simulink model "alba9b_full_loop"  (R2025b)
settings: Solver=ode15s  StartTime=0.0  StopTime=120  MaxStep=0.025  RelTol=2e-8  AbsTol=1e-9
undefined symbols (not defined in the file or in its folder): S_vec, V0_m3
settings Model: Creator=86155  LastModifiedBy=86155
settings DataIOCC: SaveFinalState=on  SaveOperatingPoint=on  SaveOutput=off  SaveState=on  SignalLogging=off  SaveTime=off

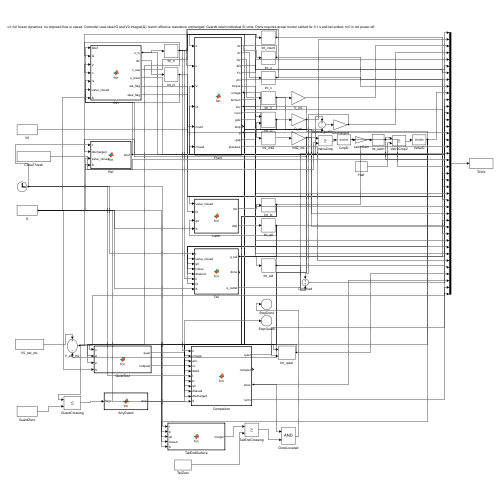
[thumbnail: Simulink's stored preview of the top-level diagram]
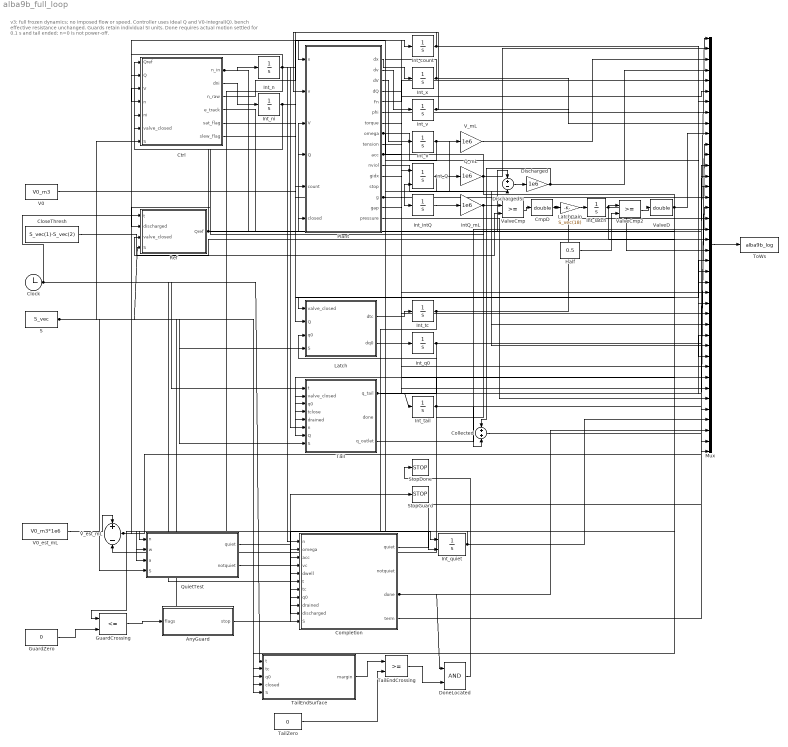
== system alba9b_full_loop ==
  note: v3: full frozen dynamics; no imposed flow or speed. Controller uses ideal Q and V0-integral(Q). bench effective resistance unchanged. Guards retain individual SI units. Done requires actual motion settled for 0.1 s and tail ended; n=0 is not power-off.
  AnyGuard : MATLAB Function  TreatAsAtomicUnit=on
  Clock : Clock
  CloseThresh : Constant  Value=S_vec(1)-S_vec(2)
  CmpD : DataTypeConversion  OutDataTypeStr=double  SaturateOnIntegerOverflow=off  RndMeth=Floor
  Collected : Sum
  Completion : MATLAB Function  TreatAsAtomicUnit=on
  Ctrl : MATLAB Function  TreatAsAtomicUnit=on
  Discharged : Gain  Gain=1e6
  DischargedSI : Sum  Inputs=+-
  DoneLocated : Logic  AllPortsSameDT=off  OutDataTypeStr=boolean
  GuardCrossing : RelationalOperator  Operator=<=  OutDataTypeStr=boolean  RndMeth=Simplest  InputSameDT=off
  GuardZero : Constant  Value=0
  Half : Constant  Value=0.5
  Int_Q : Integrator  ExternalReset=rising  AbsoluteTolerance=2e-14
  Int_V : Integrator  InitialCondition=V0_m3  AbsoluteTolerance=2e-13
  Int_count : Integrator  AbsoluteTolerance=1e-6
  Int_intQ : Integrator  AbsoluteTolerance=2e-13
  Int_latch : Integrator  LimitOutput=on  UpperSaturationLimit=1  LowerSaturationLimit=0  AbsoluteTolerance=1e-9
  Int_n : Integrator  LimitOutput=on  UpperSaturationLimit=S_vec(12)  LowerSaturationLimit=0  AbsoluteTolerance=1e-4
  Int_ni : Integrator  AbsoluteTolerance=1e-4
  Int_q0 : Integrator  AbsoluteTolerance=1e-7
  Int_quiet : Integrator  ExternalReset=rising  AbsoluteTolerance=1e-8
  Int_tail : Integrator  AbsoluteTolerance=1e-9
  Int_tc : Integrator  AbsoluteTolerance=1e-7
  Int_v : Integrator  AbsoluteTolerance=2e-10
  Int_x : Integrator  AbsoluteTolerance=2e-11
  Latch : MATLAB Function  TreatAsAtomicUnit=on
  LatchGain : Gain  Gain=S_vec(18)
  Mux : Mux  Inputs=40
  Plant : MATLAB Function  TreatAsAtomicUnit=on
  Q_mL : Gain  Gain=1e6
  QuietTest : MATLAB Function  TreatAsAtomicUnit=on
  Ref : MATLAB Function  TreatAsAtomicUnit=on
  S : Constant  Value=S_vec
  StopDone : Stop
  StopGuard : Stop
  Tail : MATLAB Function  TreatAsAtomicUnit=on
  TailEndCrossing : RelationalOperator  OutDataTypeStr=boolean  RndMeth=Simplest  InputSameDT=off
  TailEndSurface : MATLAB Function  TreatAsAtomicUnit=on
  TailZero : Constant  Value=0
  ToWs : ToWorkspace  VariableName=alba9b_log  SaveFormat=Structure With Time  SampleTime=-1
  V0 : Constant  Value=V0_m3
  V0_est_mL : Constant  Value=V0_m3*1e6
  V_est_mL : Sum  Inputs=+-
  V_mL : Gain  Gain=1e6
  ValveCmp : RelationalOperator  OutDataTypeStr=boolean  RndMeth=Simplest  InputSameDT=off
  ValveCmp2 : RelationalOperator  OutDataTypeStr=boolean  RndMeth=Simplest  InputSameDT=off
  ValveD : DataTypeConversion  OutDataTypeStr=double  SaturateOnIntegerOverflow=off  RndMeth=Floor
  intQ_mL : Gain  Gain=1e6
  wires:
  Int_x/1 -> Plant/1(x), Mux/8
  Int_v/1 -> Plant/2(v), Mux/9
  Int_V/1 -> Plant/3(V), V_mL/1, DischargedSI/2
  Int_Q/1 -> Plant/4(Q), Int_intQ/1, Q_mL/1
  Int_count/1 -> Plant/5(count), Mux/31
  ValveD/1 -> Plant/6(closed), Int_Q/2, Ref/3(valve_closed), Ctrl/6(valve_closed), Latch/1(valve_closed), Tail/2(valve_closed), Mux/10, Completion/4(vc), TailEndSurface/4(closed)
  Plant/1(dx) -> Int_x/1
  Plant/2(dv) -> Int_v/1
  Plant/3(dV) -> Int_V/1
  Plant/4(dQ) -> Int_Q/1
  Int_n/1 -> Int_count/1, Ctrl/4(n), Tail/6(n), Mux/6, Completion/1(n), QuietTest/1(n)
  Int_intQ/1 -> intQ_mL/1
  V0/1 -> DischargedSI/1
  DischargedSI/1 -> Discharged/1
  Discharged/1 -> Collected/1, Mux/4
  CloseThresh/1 -> ValveCmp/2
  ValveCmp/1 -> CmpD/1
  CmpD/1 -> LatchGain/1, Mux/21
  LatchGain/1 -> Int_latch/1
  Int_latch/1 -> ValveCmp2/1, Mux/20
  Half/1 -> ValveCmp2/2
  ValveCmp2/1 -> ValveD/1
  Clock/1 -> Ref/1(t), Tail/1(t), Completion/6(t), TailEndSurface/1(t)
  S/1 -> Ref/4(S), Ctrl/7(S), Latch/4(S), Tail/8(S), Completion/11(S), QuietTest/4(S), TailEndSurface/5(S)
  Ref/1(Qref) -> Ctrl/1(Qref), Mux/1
  Q_mL/1 -> Ctrl/2(Q), Latch/2(Q), Tail/7(Q), Mux/2
  V_mL/1 -> Mux/3
  Int_ni/1 -> Ctrl/5(ni), Mux/16
  Ctrl/1(n_in) -> Int_n/1, Mux/15
  Ctrl/2(dni) -> Int_ni/1
  Int_q0/1 -> Latch/3(q0), Tail/3(q0), Mux/17, Completion/8(q0), TailEndSurface/3(q0)
  Latch/1(dtc) -> Int_tc/1
  Latch/2(dq0) -> Int_q0/1
  Int_tc/1 -> Tail/4(tclose), Mux/18, Completion/7(tc), TailEndSurface/2(tc)
  Int_tail/1 -> Tail/5(drained), Collected/2, Mux/12, Completion/9(drained)
  Tail/1(q_tail) -> Int_tail/1, Mux/11
  Plant/5(Fn) -> Mux/5
  Ctrl/3(n_raw) -> Mux/7
  Collected/1 -> Mux/13
  Ctrl/4(e_track) -> Mux/14
  Tail/3(q_outlet) -> Mux/19
  Ctrl/5(sat_flag) -> Mux/22
  Ctrl/6(slew_flag) -> Mux/23
  Plant/6(phi) -> Mux/24
  Plant/7(torque) -> Mux/25
  Plant/8(omega) -> Mux/26, Completion/2(omega), QuietTest/2(w)
  Plant/9(tension) -> Mux/27
  Plant/11(nviol) -> Mux/28
  Plant/12(gidx) -> Mux/29
  intQ_mL/1 -> Mux/30, V_est_mL/2, Ref/2(discharged), ValveCmp/1, Completion/10(discharged)
  Plant/10(acc) -> Mux/32, Completion/3(acc), QuietTest/3(a)
  Mux/1 -> ToWs/1
  V0_est_mL/1 -> V_est_mL/1
  V_est_mL/1 -> Ctrl/3(V), Mux/36
  Int_quiet/1 -> Completion/5(dwell), Mux/37
  QuietTest/1(quiet) -> Int_quiet/1
  QuietTest/2(notquiet) -> Int_quiet/2
  TailEndSurface/1(margin) -> TailEndCrossing/1
  TailZero/1 -> TailEndCrossing/2
  Completion/3(done) -> DoneLocated/1, Mux/38
  TailEndCrossing/1 -> DoneLocated/2
  DoneLocated/1 -> StopDone/1
  Plant/14(g) -> GuardCrossing/1, Mux/33
  GuardZero/1 -> GuardCrossing/2
  GuardCrossing/1 -> AnyGuard/1(flags)
  AnyGuard/1(stop) -> StopGuard/1
  Plant/15(gap) -> Mux/34
  Plant/16(pressure) -> Mux/35
  Completion/4(term) -> Mux/39
  Completion/1(quiet) -> Mux/40

== matlab function alba9b_full_loop/Completion ==
  data: n input; quiet output; omega input; acc input; vc input; dwell input; t input; tc input; q0 input; drained input; discharged input; S input; notquiet output; done output; term output
function [quiet,notquiet,done,term] = fcn(n,omega,acc,vc,dwell,t,tc,q0,drained,discharged,S)
%#codegen
quiet=double(abs(n)<=S(22) && abs(omega)<=S(23) && abs(acc)<=S(24));
notquiet=1-quiet;
T=inf; if q0>0, T=2*S(3)/q0; end
done=double(vc>0.5 && t>=tc+T && drained>=S(3)-1e-6 && dwell>=S(25));
term=double(S(20)>0.5 && S(1)-S(2)-discharged<=S(21));
end

== matlab function alba9b_full_loop/QuietTest ==
  data: n input; quiet output; w input; a input; S input; notquiet output
function [quiet,notquiet]=fcn(n,w,a,S)
%#codegen
quiet=double(abs(n)<=S(22) && abs(w)<=S(23) && abs(a)<=S(24));
notquiet=1-quiet;
end

== matlab function alba9b_full_loop/TailEndSurface ==
  data: t input; margin output; tc input; q0 input; closed input; S input
function margin=fcn(t,tc,q0,closed,S)
%#codegen
margin=-1; if closed>0.5 && q0>0, margin=t-tc-2*S(3)/q0; end
end

== matlab function alba9b_full_loop/AnyGuard ==
  data: flags input; stop output
function stop=fcn(flags)
%#codegen
stop=any(flags);
end

== matlab function alba9b_full_loop/Ctrl ==
  data: Qref input; n_in output; Q input; V input; n input; ni input; valve_closed input; S input; dni output; n_raw output; e_track output; sat_flag output; slew_flag output
function [n_in,dni,n_raw,e_track,sat_flag,slew_flag] = fcn(Qref,Q,V,n,ni,valve_closed,S)
%#codegen
% identical to model A: same gains, same structure, no retuning in stage B
[n_in,dni,n_raw,e_track,~,sat_flag,slew_flag] = ...
    alba9_controller(Qref,Q,V,n,ni,valve_closed,S);

== matlab function alba9b_full_loop/Ref ==
  data: t input; Qref output; discharged input; valve_closed input; S input
function Qref = fcn(t,discharged,valve_closed,S)
%#codegen
Qref = alba9_reference(t,discharged,valve_closed,S);

== matlab function alba9b_full_loop/Plant ==
  data: x input; dx output; v input; V input; Q input; count input; closed input; dv output; dV output; dQ output; Fn output; phi output; torque output; omega output; tension output; acc output; nviol output; gidx output; stop output; g output; gap output; pressure output
function [dx,dv,dV,dQ,Fn,phi,torque,omega,tension,acc,nviol,gidx,stop,g,gap,pressure] = fcn(x,v,V,Q,count,closed)
%#codegen
[dx,dv,dV,dQ,Fn,phi,torque,omega,tension,acc,nviol,gidx,stop,g,gap,pressure]=alba9b_plant_block(x,v,V,Q,count,closed);
end

== matlab function alba9b_full_loop/Latch ==
  data: valve_closed input; dtc output; Q input; q0 input; S input; dq0 output
function [dtc,dq0] = fcn(valve_closed,Q,q0,S)
%#codegen
isopen = 1 - min(max(valve_closed,0),1);
dtc = isopen;
dq0 = isopen*(Q-q0)/S(19);

== matlab function alba9b_full_loop/Tail ==
  data: t input; q_tail output; valve_closed input; q0 input; tclose input; drained input; n input; Q input; S input; done output; q_outlet output
function [q_tail,done,q_outlet] = fcn(t,valve_closed,q0,tclose,drained,n,Q,S)
%#codegen
[q_tail,done,q_outlet] = alba9_tail(t,valve_closed,q0,tclose,drained,n,Q,S);
